simulink model "xpccan104fifo1"  (Simulink 6.0)
settings: Solver=FixedStepDiscrete  StartTime=0.0  StopTime=inf  RelTol=1e-3
libraries: xpclib x12, simulink x1
settings Model: Creator=mvetsch  LastModifiedBy=ekbas  ExtModeArmWhenConnect=off  BufferReuse=off  SignalLoggingName=logsOut  BlockReductionOpt=off  OptimizeBlockIOStorage=off  ZeroCrossControl=UseLocalSettings  ProdHWDeviceType=Microprocessor  TargetHWChar=2  TargetHWWordLengths=8,16,32,32  RTWSystemTargetFile=xpctarget.tlc  RTWTemplateMakefile=xpc_default_tmf  RTWMathFcnLibMatFile=iso_c_tmw.mat  RTWOptions="-aEnforceIntegerDowncast=1 -aFoldNonRolledExpr=1 -aInlineInvariantSignals=0 -aInlineParameters=0 -aLocalBlockOutputs=0 -aRollThreshold=5 -aGenerateReport=0 -aGenCodeOnly=0 -aRTWVerbose=1 -aForceParamTrailComments=0 -aGenerateComments=1 -aIgnoreCustomStorageClasses=1 -aIncHierarchyInIds=0 -aMaxRTWIdLen=31 -aShowEliminatedStatements=1 -aPrefixModelToSubsysFcnNames=1 -aIncDataTypeInIds=0 -aInlinedPrmAccess=\"Literals\" -aTargetFcnLib=\"iso_c_tmw.mat\" -aGenerateFullHeader=1 -aIsPILTarget=0 -aRL32ModeModifier=\"Real-Time\" -aRL32LogTETModifier=1 -aRL32LogBufSizeModifier=100000 -aRL32IRQSourceModifier=\"Timer\" -axPCIRQSourceBoard=\"None/Other\" -axPCIOIRQSlot=-1 -axpcDblBuff=0 -axpcObjCom=0 -aRL32ObjectName=\"tg\" -aExtMode=1 -aRL32ScopeModifier=1"  SimulationMode=external
settings ConfigSet: SimulationMode=external
settings DataIOCC: SignalLoggingName=logsOut
settings OptimizationCC: BlockReduction=off  BooleanDataType=off  InlineInvariantSignals=off  OptimizeBlockIOStorage=off  BufferReuse=off  LocalBlockOutputs=off  MultiInstanced=off
settings FormatCC: IgnoreBidirectionalLines=off
settings HardwareCC: ProdHWDeviceType=Microprocessor  ShiftRightIntArith=on  TargetHWCharacteristics=InheritFromRTWHook
settings RTWCC: SystemTargetFile=xpctarget.tlc  TemplateMakefile=xpc_default_tmf  ProcessScript=xpctarget_make_rtw_hook
settings CodeAppCC: FileBanners=off
settings STFCustomTargetCC: TargetFcnLib=iso_c_tmw.mat  IsERTTarget=off  SystemTargetFile=xpctarget.tlc
settings CustomProperty: DataType=RTWOptions_EnumType_D__Axpc_matlab_toolbox_rtw_targets_xpc_xpc_xpctarget_RL32ModeModifier  Value=Real-Time
settings EnumStrPairs: String=Real-Time

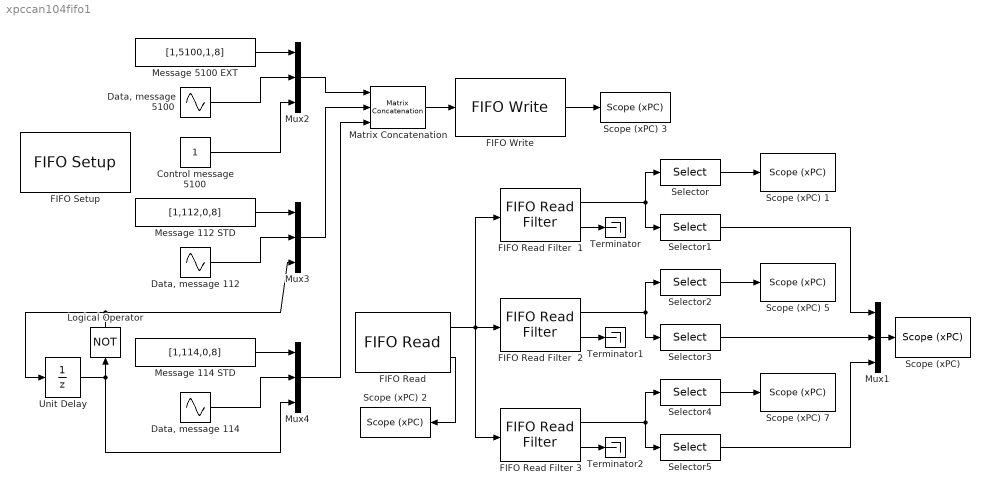
== system xpccan104fifo1 ==
  Control message 5100 : Constant  VectorParams1D=off
  "Data, message 112" : Sin  Amplitude=2  Frequency=20*2*pi  SampleTime=0.001
  "Data, message 114" : Sin  Amplitude=3  Frequency=20*2*pi  SampleTime=0.001
  "Data, message 5100" : Sin  Frequency=20*2*pi  SampleTime=0.001
  "FIFO Read " : xpclib/CAN/Softing/CAN-AC2-104 SJA 1000/FIFO Mode/FIFO Read   board=1  depth=3  status=on  sampletime=0.001
  FIFO Read Filter  1 : xpclib/CAN/Softing/CAN-AC2-PCI SJA 1000/FIFO Mode/FIFO Read Filter   portin=2  ctypein=EDF  direction=Include  ident=[5100]  identsel=Include
  FIFO Read Filter  2 : xpclib/CAN/Softing/CAN-AC2-PCI SJA 1000/FIFO Mode/FIFO Read Filter   portin=2  ctypein=SDF  direction=Include  ident=[112]  identsel=Include
  FIFO Read Filter 3 : xpclib/CAN/Softing/CAN-AC2-PCI SJA 1000/FIFO Mode/FIFO Read Filter   portin=2  ctypein=SDF  direction=Include  ident=[114]  identsel=Include
  "FIFO Setup " : xpclib/CAN/Softing/CAN-AC2-104 SJA 1000/FIFO Mode/FIFO Setup   board=1  can1Baudrate=1 MBaud  can1UserBR=[1,1,4,3]  acc1=[0,0,0,0]  can2Baudrate=1 MBaud  can2UserBR=[1,1,4,3]  acc2=[0,0,0,0]  efdetection=off  init=[]  term=[]  ioBaseAddressL=0x300  memBaseAddressL=0xd0000  intNo=None
  "FIFO Write " : xpclib/CAN/Softing/CAN-AC2-104 SJA 1000/FIFO Mode/FIFO Write   board=1  status=on  sampletime=-1
  Logical Operator : Logic  Orientation=up  Operator=NOT
  Matrix Concatenation : simulink/Math Operations/Matrix Concatenation  numInports=3  catMethod=Vertical
  Message 112 STD : Constant  Value=[1,112,0,8]  VectorParams1D=off
  Message 114 STD : Constant  Value=[1,114,0,8]  VectorParams1D=off
  Message 5100 EXT : Constant  Value=[1,5100,1,8]  VectorParams1D=off
  Mux{1..4} (4 alike) : Mux  Inputs=3
  "Scope (xPC) " : xpclib/Misc./Scope (xPC)   scopeno=3  scopetype=Target  autostart=on  viewmode=Graphical redraw  formatstr='%15.6f'  grid=on  ylimits=[0,0]  nosamples=100  noprepostsamples=0  interleave=1  triggermode=FreeRun  triggersignal=1  triggerlevel=0.0  triggerslope=Either  triggerscope=1  triggersample=0  filename=data.dat  mode=Lazy  writesize=512  autorestart=off
  Scope (xPC) 1 : xpclib/Misc./Scope (xPC)   scopeno=4  scopetype=Target  autostart=on  viewmode=Numerical  formatstr='%15.6f'  grid=on  ylimits=[0,0]  nosamples=3  noprepostsamples=0  interleave=1  triggermode=FreeRun  triggersignal=1  triggerlevel=0.0  triggerslope=Either  triggerscope=1  triggersample=0  filename=data.dat  mode=Lazy  writesize=512  autorestart=off
  Scope (xPC) 2 : xpclib/Misc./Scope (xPC)   Orientation=left  scopeno=2  scopetype=Target  autostart=on  viewmode=Numerical  formatstr='%15.6f'  grid=on  ylimits=[0,0]  nosamples=3  noprepostsamples=0  interleave=1  triggermode=FreeRun  triggersignal=1  triggerlevel=0.0  triggerslope=Either  triggerscope=1  triggersample=0  filename=data.dat  mode=Lazy  writesize=512  autorestart=off
  Scope (xPC) 3 : xpclib/Misc./Scope (xPC)   scopeno=1  scopetype=Target  autostart=on  viewmode=Numerical  formatstr='%15.6f'  grid=on  ylimits=[0,0]  nosamples=3  noprepostsamples=0  interleave=1  triggermode=FreeRun  triggersignal=1  triggerlevel=0.0  triggerslope=Either  triggerscope=1  triggersample=0  filename=data.dat  mode=Lazy  writesize=512  autorestart=off
  Scope (xPC) 5 : xpclib/Misc./Scope (xPC)   scopeno=5  scopetype=Target  autostart=on  viewmode=Numerical  formatstr='%15.6f'  grid=on  ylimits=[0,0]  nosamples=3  noprepostsamples=0  interleave=1  triggermode=FreeRun  triggersignal=1  triggerlevel=0.0  triggerslope=Either  triggerscope=1  triggersample=0  filename=data.dat  mode=Lazy  writesize=512  autorestart=off
  Scope (xPC) 7 : xpclib/Misc./Scope (xPC)   scopeno=6  scopetype=Target  autostart=on  viewmode=Numerical  formatstr='%15.6f'  grid=on  ylimits=[0,0]  nosamples=3  noprepostsamples=0  interleave=1  triggermode=FreeRun  triggersignal=1  triggerlevel=0.0  triggerslope=Either  triggerscope=1  triggersample=0  filename=data.dat  mode=Lazy  writesize=512  autorestart=off
  Selector : Selector  Elements=[1:5]  InputPortWidth=6
  Selector1 : Selector  Elements=[6]  InputPortWidth=6
  Selector2 : Selector  Elements=[1:5]  InputPortWidth=6
  Selector3 : Selector  Elements=[6]  InputPortWidth=6
  Selector4 : Selector  Elements=[1:5]  InputPortWidth=6
  Selector5 : Selector  Elements=[6]  InputPortWidth=6
  Terminator : Terminator
  Terminator1 : Terminator
  Terminator2 : Terminator
  Unit Delay : UnitDelay  SampleTime=0.001
  wires:
  Message 5100 EXT/1 -> Mux2/1
  "Data, message 5100"/1 -> Mux2/2
  "FIFO Read "/1 -> FIFO Read Filter  1/1, FIFO Read Filter  2/1, FIFO Read Filter 3/1
  "FIFO Read "/2 -> Scope (xPC) 2/1
  "FIFO Write "/1 -> Scope (xPC) 3/1
  Control message 5100/1 -> Mux2/3
  Unit Delay/1 -> Logical Operator/1, Mux4/3
  Logical Operator/1 -> Unit Delay/1, Mux3/3
  Message 112 STD/1 -> Mux3/1
  "Data, message 112"/1 -> Mux3/2
  Message 114 STD/1 -> Mux4/1
  "Data, message 114"/1 -> Mux4/2
  Mux3/1 -> Matrix Concatenation/2
  Mux2/1 -> Matrix Concatenation/1
  Mux4/1 -> Matrix Concatenation/3
  Matrix Concatenation/1 -> "FIFO Write "/1
  FIFO Read Filter  1/1 -> Selector/1, Selector1/1
  Selector/1 -> Scope (xPC) 1/1
  Selector2/1 -> Scope (xPC) 5/1
  Selector3/1 -> Mux1/2
  FIFO Read Filter  2/1 -> Selector2/1, Selector3/1
  Selector4/1 -> Scope (xPC) 7/1
  Selector5/1 -> Mux1/3
  FIFO Read Filter 3/1 -> Selector4/1, Selector5/1
  FIFO Read Filter  1/2 -> Terminator/1
  FIFO Read Filter  2/2 -> Terminator1/1
  FIFO Read Filter 3/2 -> Terminator2/1
  Selector1/1 -> Mux1/1
  Mux1/1 -> "Scope (xPC) "/1
